simulink model "raio_calculo"  (R2023a)
settings: Solver=VariableStepAuto  StartTime=0.0  StopTime=10.0  RelTol=1e-3
settings Model: Creator=thailon  LastModifiedBy=thailon
settings RTWCC: GPUComputeCapability=5.0
settings ConfigComp: CovBoundaryAbsTol=1.0e-5

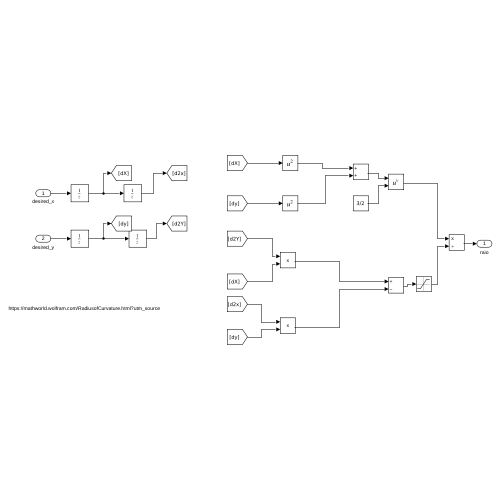
[thumbnail: Simulink's stored preview of the top-level diagram]
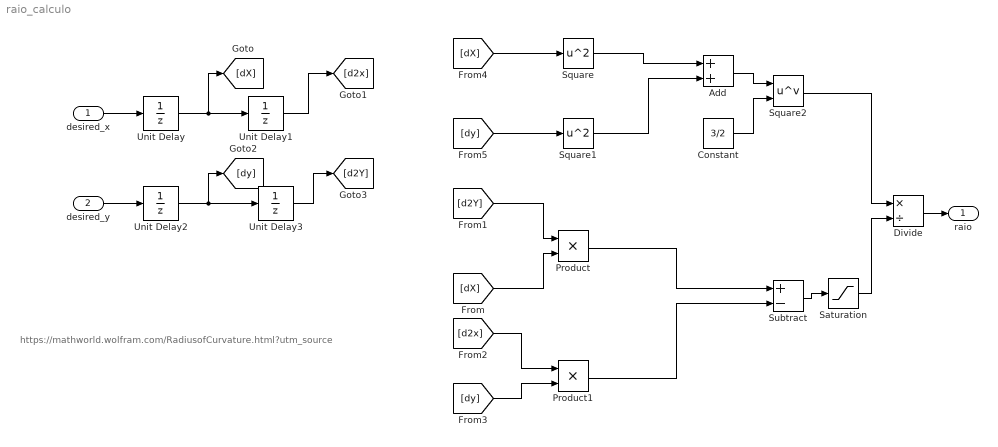
== system raio_calculo ==
  note: https://mathworld.wolfram.com/RadiusofCurvature.html?utm_source
  desired_x : Inport
  desired_y : Inport  Port=2
  Add : Sum
  Constant : Constant  Value=3/2
  Divide : Product  Inputs=*/
  Product : Product
  Product1 : Product
  Saturation : Saturate  UpperLimit=10000  LowerLimit=0.00001
  Square : Math  Operator=square
  Square1 : Math  Operator=square
  Square2 : Math  Operator=pow
  Subtract : Sum  Inputs=+-
  Unit Delay{,1..3} (4 alike) : UnitDelay  SampleTime=-1  HasFrameUpgradeWarning=on
  raio : Outport
  wires:
  desired_x/1 -> Unit Delay/1
  Unit Delay/1 -> [dX], Unit Delay1/1
  desired_y/1 -> Unit Delay2/1
  Unit Delay2/1 -> [dy], Unit Delay3/1
  Unit Delay1/1 -> [d2x]
  Unit Delay3/1 -> [d2Y]
  [dX] -> Product/2
  [d2Y] -> Product/1
  Product/1 -> Subtract/1
  [d2x] -> Product1/1
  [dy] -> Product1/2
  Product1/1 -> Subtract/2
  [dX] -> Square/1
  [dy] -> Square1/1
  Square1/1 -> Add/2
  Square/1 -> Add/1
  Add/1 -> Square2/1
  Constant/1 -> Square2/2
  Divide/1 -> raio/1
  Square2/1 -> Divide/1
  Subtract/1 -> Saturation/1
  Saturation/1 -> Divide/2
